simulink model "HybridControllerD3D3"  (Simulink 7.5)
settings: Solver=FixedStepDiscrete  StartTime=0.0  StopTime=inf  FixedStep=samplePeriod  RelTol=1e-3  AbsTol=1e-6
PreLoadFcn:
  | initializeSimulation;
InitFcn:
  | clear('all');
  | initializeSimulation;
undefined symbols (not defined in the file): damperA, damperB, damperC, damperCanon, DiscIntNeverNeededParam, flowCanon, forceCanon, frictionA, frictionB, frictionC, gasConstant, HybridCtrlParameters, lengthCanon, massA, massB, massC, massCanon, maxDisplA, maxDisplB, maxDisplC, maxOilVolume, maxVelocA, maxVelocB, maxVelocC, minDisplA, minDisplB, minDisplC, minVelocA, minVelocB, minVelocC, nAct, nAdcU, nDinp, nDout, nDucU, nEncU, precharge, pumpFlow, returnPress, staticForceA, staticForceB, staticForceC, supplyPress, velocCanon, volume, volumeCanon, yieldDisplA, yieldDisplB, yieldDisplC
libraries: simulink x2
(part 3 of 3)

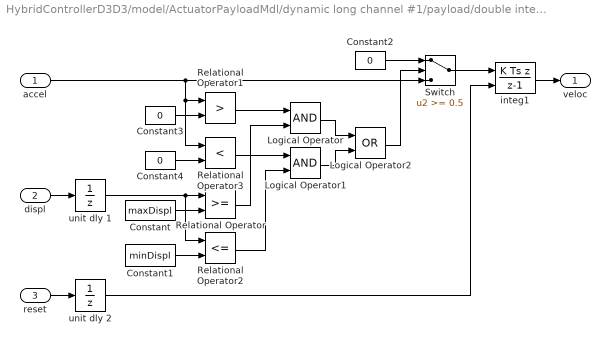
== system HybridControllerD3D3/model/ActuatorPayloadMdl/dynamic long channel #1/payload/double integrator/veloc gen ==
  accel : Inport  OutDataType=sfix(16)  OutScaling=2^0
  displ : Inport  Port=2  OutDataType=sfix(16)  OutScaling=2^0
  reset : Inport  Port=3  OutDataType=sfix(16)  OutScaling=2^0
  Constant : Constant  Value=maxDispl  OutDataType=sfix(16)  OutScaling=2^0
  Constant1 : Constant  Value=minDispl  OutDataType=sfix(16)  OutScaling=2^0
  Constant2 : Constant  Value=0  OutDataType=sfix(16)  OutScaling=2^0
  Constant3 : Constant  Value=0  OutDataType=sfix(16)  OutScaling=2^0
  Constant4 : Constant  Value=0  OutDataType=sfix(16)  OutScaling=2^0
  Logical Operator : Logic
  Logical Operator1 : Logic
  Logical Operator2 : Logic  Operator=OR
  Relational Operator : RelationalOperator  InputSameDT=on
  Relational Operator1 : RelationalOperator  Operator=>  InputSameDT=on
  Relational Operator2 : RelationalOperator  Operator=<=  InputSameDT=on
  Relational Operator3 : RelationalOperator  Operator=<  InputSameDT=on
  Switch : Switch  Threshold=0.5  SaturateOnIntegerOverflow=on  InputSameDT=on
  integ1 : DiscreteIntegrator  IntegratorMethod=Integration: Backward Euler  ExternalReset=either  SampleTime=-1  OutDataType=sfix(16)  OutScaling=2^0  LimitOutput=on  UpperSaturationLimit=maxVeloc  LowerSaturationLimit=minVeloc  ICPrevOutput=DiscIntNeverNeededParam  ICPrevScaledInput=DiscIntNeverNeededParam
  unit dly 1 : UnitDelay  SampleTime=-1
  unit dly 2 : UnitDelay  SampleTime=-1
  veloc : Outport  OutDataType=sfix(16)  OutScaling=2^0
  wires:
  unit dly 1/1 -> Relational Operator2/1, Relational Operator/1
  reset/1 -> unit dly 2/1
  displ/1 -> unit dly 1/1
  Logical Operator1/1 -> Logical Operator2/2
  unit dly 2/1 -> integ1/2
  Switch/1 -> integ1/1
  Logical Operator2/1 -> Switch/2
  Constant2/1 -> Switch/1
  Logical Operator/1 -> Logical Operator2/1
  Relational Operator3/1 -> Logical Operator1/1
  Constant4/1 -> Relational Operator3/2
  Relational Operator1/1 -> Logical Operator/1
  Constant3/1 -> Relational Operator1/2
  accel/1 -> Switch/3, Relational Operator1/1, Relational Operator3/1
  Constant1/1 -> Relational Operator2/2
  Relational Operator2/1 -> Logical Operator1/2
  Relational Operator/1 -> Logical Operator/2
  Constant/1 -> Relational Operator/2
  integ1/1 -> veloc/1

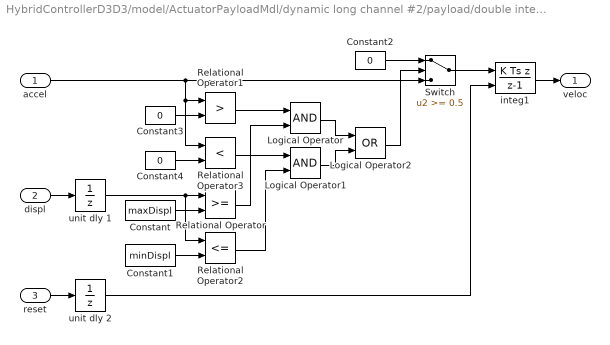
== system HybridControllerD3D3/model/ActuatorPayloadMdl/dynamic long channel #2/payload/double integrator/veloc gen ==
  accel : Inport  OutDataType=sfix(16)  OutScaling=2^0
  displ : Inport  Port=2  OutDataType=sfix(16)  OutScaling=2^0
  reset : Inport  Port=3  OutDataType=sfix(16)  OutScaling=2^0
  Constant : Constant  Value=maxDispl  OutDataType=sfix(16)  OutScaling=2^0
  Constant1 : Constant  Value=minDispl  OutDataType=sfix(16)  OutScaling=2^0
  Constant2 : Constant  Value=0  OutDataType=sfix(16)  OutScaling=2^0
  Constant3 : Constant  Value=0  OutDataType=sfix(16)  OutScaling=2^0
  Constant4 : Constant  Value=0  OutDataType=sfix(16)  OutScaling=2^0
  Logical Operator : Logic
  Logical Operator1 : Logic
  Logical Operator2 : Logic  Operator=OR
  Relational Operator : RelationalOperator  InputSameDT=on
  Relational Operator1 : RelationalOperator  Operator=>  InputSameDT=on
  Relational Operator2 : RelationalOperator  Operator=<=  InputSameDT=on
  Relational Operator3 : RelationalOperator  Operator=<  InputSameDT=on
  Switch : Switch  Threshold=0.5  SaturateOnIntegerOverflow=on  InputSameDT=on
  integ1 : DiscreteIntegrator  IntegratorMethod=Integration: Backward Euler  ExternalReset=either  SampleTime=-1  OutDataType=sfix(16)  OutScaling=2^0  LimitOutput=on  UpperSaturationLimit=maxVeloc  LowerSaturationLimit=minVeloc  ICPrevOutput=DiscIntNeverNeededParam  ICPrevScaledInput=DiscIntNeverNeededParam
  unit dly 1 : UnitDelay  SampleTime=-1
  unit dly 2 : UnitDelay  SampleTime=-1
  veloc : Outport  OutDataType=sfix(16)  OutScaling=2^0
  wires:
  unit dly 1/1 -> Relational Operator2/1, Relational Operator/1
  reset/1 -> unit dly 2/1
  displ/1 -> unit dly 1/1
  Logical Operator1/1 -> Logical Operator2/2
  unit dly 2/1 -> integ1/2
  Switch/1 -> integ1/1
  Logical Operator2/1 -> Switch/2
  Constant2/1 -> Switch/1
  Logical Operator/1 -> Logical Operator2/1
  Relational Operator3/1 -> Logical Operator1/1
  Constant4/1 -> Relational Operator3/2
  Relational Operator1/1 -> Logical Operator/1
  Constant3/1 -> Relational Operator1/2
  accel/1 -> Switch/3, Relational Operator1/1, Relational Operator3/1
  Constant1/1 -> Relational Operator2/2
  Relational Operator2/1 -> Logical Operator1/2
  Relational Operator/1 -> Logical Operator/2
  Constant/1 -> Relational Operator/2
  integ1/1 -> veloc/1

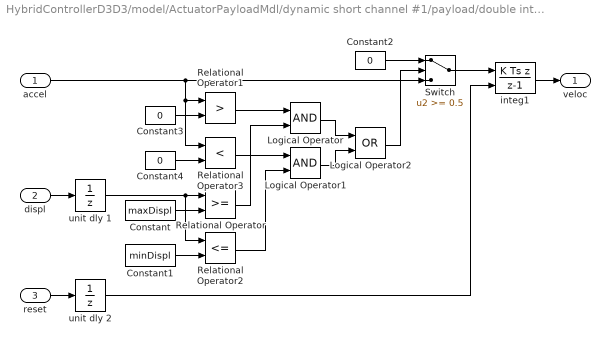
== system HybridControllerD3D3/model/ActuatorPayloadMdl/dynamic short channel #1/payload/double integrator/veloc gen ==
  accel : Inport  OutDataType=sfix(16)  OutScaling=2^0
  displ : Inport  Port=2  OutDataType=sfix(16)  OutScaling=2^0
  reset : Inport  Port=3  OutDataType=sfix(16)  OutScaling=2^0
  Constant : Constant  Value=maxDispl  OutDataType=sfix(16)  OutScaling=2^0
  Constant1 : Constant  Value=minDispl  OutDataType=sfix(16)  OutScaling=2^0
  Constant2 : Constant  Value=0  OutDataType=sfix(16)  OutScaling=2^0
  Constant3 : Constant  Value=0  OutDataType=sfix(16)  OutScaling=2^0
  Constant4 : Constant  Value=0  OutDataType=sfix(16)  OutScaling=2^0
  Logical Operator : Logic
  Logical Operator1 : Logic
  Logical Operator2 : Logic  Operator=OR
  Relational Operator : RelationalOperator  InputSameDT=on
  Relational Operator1 : RelationalOperator  Operator=>  InputSameDT=on
  Relational Operator2 : RelationalOperator  Operator=<=  InputSameDT=on
  Relational Operator3 : RelationalOperator  Operator=<  InputSameDT=on
  Switch : Switch  Threshold=0.5  SaturateOnIntegerOverflow=on  InputSameDT=on
  integ1 : DiscreteIntegrator  IntegratorMethod=Integration: Backward Euler  ExternalReset=either  SampleTime=-1  OutDataType=sfix(16)  OutScaling=2^0  LimitOutput=on  UpperSaturationLimit=maxVeloc  LowerSaturationLimit=minVeloc  ICPrevOutput=DiscIntNeverNeededParam  ICPrevScaledInput=DiscIntNeverNeededParam
  unit dly 1 : UnitDelay  SampleTime=-1
  unit dly 2 : UnitDelay  SampleTime=-1
  veloc : Outport  OutDataType=sfix(16)  OutScaling=2^0
  wires:
  unit dly 1/1 -> Relational Operator2/1, Relational Operator/1
  reset/1 -> unit dly 2/1
  displ/1 -> unit dly 1/1
  Logical Operator1/1 -> Logical Operator2/2
  unit dly 2/1 -> integ1/2
  Switch/1 -> integ1/1
  Logical Operator2/1 -> Switch/2
  Constant2/1 -> Switch/1
  Logical Operator/1 -> Logical Operator2/1
  Relational Operator3/1 -> Logical Operator1/1
  Constant4/1 -> Relational Operator3/2
  Relational Operator1/1 -> Logical Operator/1
  Constant3/1 -> Relational Operator1/2
  accel/1 -> Switch/3, Relational Operator1/1, Relational Operator3/1
  Constant1/1 -> Relational Operator2/2
  Relational Operator2/1 -> Logical Operator1/2
  Relational Operator/1 -> Logical Operator/2
  Constant/1 -> Relational Operator/2
  integ1/1 -> veloc/1

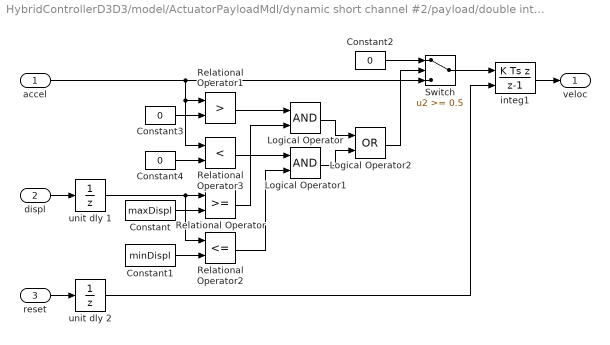
== system HybridControllerD3D3/model/ActuatorPayloadMdl/dynamic short channel #2/payload/double integrator/veloc gen ==
  accel : Inport  OutDataType=sfix(16)  OutScaling=2^0
  displ : Inport  Port=2  OutDataType=sfix(16)  OutScaling=2^0
  reset : Inport  Port=3  OutDataType=sfix(16)  OutScaling=2^0
  Constant : Constant  Value=maxDispl  OutDataType=sfix(16)  OutScaling=2^0
  Constant1 : Constant  Value=minDispl  OutDataType=sfix(16)  OutScaling=2^0
  Constant2 : Constant  Value=0  OutDataType=sfix(16)  OutScaling=2^0
  Constant3 : Constant  Value=0  OutDataType=sfix(16)  OutScaling=2^0
  Constant4 : Constant  Value=0  OutDataType=sfix(16)  OutScaling=2^0
  Logical Operator : Logic
  Logical Operator1 : Logic
  Logical Operator2 : Logic  Operator=OR
  Relational Operator : RelationalOperator  InputSameDT=on
  Relational Operator1 : RelationalOperator  Operator=>  InputSameDT=on
  Relational Operator2 : RelationalOperator  Operator=<=  InputSameDT=on
  Relational Operator3 : RelationalOperator  Operator=<  InputSameDT=on
  Switch : Switch  Threshold=0.5  SaturateOnIntegerOverflow=on  InputSameDT=on
  integ1 : DiscreteIntegrator  IntegratorMethod=Integration: Backward Euler  ExternalReset=either  SampleTime=-1  OutDataType=sfix(16)  OutScaling=2^0  LimitOutput=on  UpperSaturationLimit=maxVeloc  LowerSaturationLimit=minVeloc  ICPrevOutput=DiscIntNeverNeededParam  ICPrevScaledInput=DiscIntNeverNeededParam
  unit dly 1 : UnitDelay  SampleTime=-1
  unit dly 2 : UnitDelay  SampleTime=-1
  veloc : Outport  OutDataType=sfix(16)  OutScaling=2^0
  wires:
  unit dly 1/1 -> Relational Operator2/1, Relational Operator/1
  reset/1 -> unit dly 2/1
  displ/1 -> unit dly 1/1
  Logical Operator1/1 -> Logical Operator2/2
  unit dly 2/1 -> integ1/2
  Switch/1 -> integ1/1
  Logical Operator2/1 -> Switch/2
  Constant2/1 -> Switch/1
  Logical Operator/1 -> Logical Operator2/1
  Relational Operator3/1 -> Logical Operator1/1
  Constant4/1 -> Relational Operator3/2
  Relational Operator1/1 -> Logical Operator/1
  Constant3/1 -> Relational Operator1/2
  accel/1 -> Switch/3, Relational Operator1/1, Relational Operator3/1
  Constant1/1 -> Relational Operator2/2
  Relational Operator2/1 -> Logical Operator1/2
  Relational Operator/1 -> Logical Operator/2
  Constant/1 -> Relational Operator/2
  integ1/1 -> veloc/1

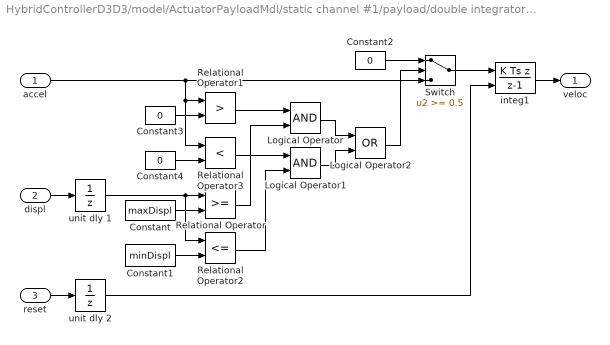
== system HybridControllerD3D3/model/ActuatorPayloadMdl/static channel #1/payload/double integrator/veloc gen ==
  accel : Inport  OutDataType=sfix(16)  OutScaling=2^0
  displ : Inport  Port=2  OutDataType=sfix(16)  OutScaling=2^0
  reset : Inport  Port=3  OutDataType=sfix(16)  OutScaling=2^0
  Constant : Constant  Value=maxDispl  OutDataType=sfix(16)  OutScaling=2^0
  Constant1 : Constant  Value=minDispl  OutDataType=sfix(16)  OutScaling=2^0
  Constant2 : Constant  Value=0  OutDataType=sfix(16)  OutScaling=2^0
  Constant3 : Constant  Value=0  OutDataType=sfix(16)  OutScaling=2^0
  Constant4 : Constant  Value=0  OutDataType=sfix(16)  OutScaling=2^0
  Logical Operator : Logic
  Logical Operator1 : Logic
  Logical Operator2 : Logic  Operator=OR
  Relational Operator : RelationalOperator  InputSameDT=on
  Relational Operator1 : RelationalOperator  Operator=>  InputSameDT=on
  Relational Operator2 : RelationalOperator  Operator=<=  InputSameDT=on
  Relational Operator3 : RelationalOperator  Operator=<  InputSameDT=on
  Switch : Switch  Threshold=0.5  SaturateOnIntegerOverflow=on  InputSameDT=on
  integ1 : DiscreteIntegrator  IntegratorMethod=Integration: Backward Euler  ExternalReset=either  SampleTime=-1  OutDataType=sfix(16)  OutScaling=2^0  LimitOutput=on  UpperSaturationLimit=maxVeloc  LowerSaturationLimit=minVeloc  ICPrevOutput=DiscIntNeverNeededParam  ICPrevScaledInput=DiscIntNeverNeededParam
  unit dly 1 : UnitDelay  SampleTime=-1
  unit dly 2 : UnitDelay  SampleTime=-1
  veloc : Outport  OutDataType=sfix(16)  OutScaling=2^0
  wires:
  unit dly 1/1 -> Relational Operator2/1, Relational Operator/1
  reset/1 -> unit dly 2/1
  displ/1 -> unit dly 1/1
  Logical Operator1/1 -> Logical Operator2/2
  unit dly 2/1 -> integ1/2
  Switch/1 -> integ1/1
  Logical Operator2/1 -> Switch/2
  Constant2/1 -> Switch/1
  Logical Operator/1 -> Logical Operator2/1
  Relational Operator3/1 -> Logical Operator1/1
  Constant4/1 -> Relational Operator3/2
  Relational Operator1/1 -> Logical Operator/1
  Constant3/1 -> Relational Operator1/2
  accel/1 -> Switch/3, Relational Operator1/1, Relational Operator3/1
  Constant1/1 -> Relational Operator2/2
  Relational Operator2/1 -> Logical Operator1/2
  Relational Operator/1 -> Logical Operator/2
  Constant/1 -> Relational Operator/2
  integ1/1 -> veloc/1

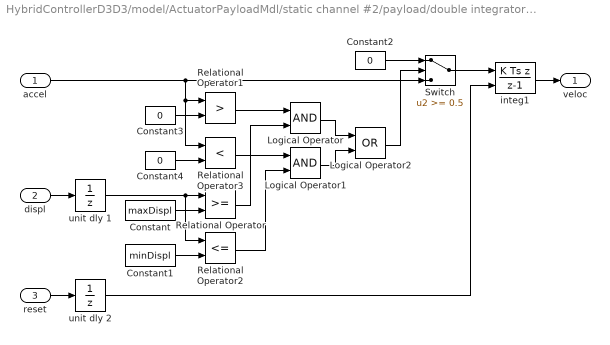
== system HybridControllerD3D3/model/ActuatorPayloadMdl/static channel #2/payload/double integrator/veloc gen ==
  accel : Inport  OutDataType=sfix(16)  OutScaling=2^0
  displ : Inport  Port=2  OutDataType=sfix(16)  OutScaling=2^0
  reset : Inport  Port=3  OutDataType=sfix(16)  OutScaling=2^0
  Constant : Constant  Value=maxDispl  OutDataType=sfix(16)  OutScaling=2^0
  Constant1 : Constant  Value=minDispl  OutDataType=sfix(16)  OutScaling=2^0
  Constant2 : Constant  Value=0  OutDataType=sfix(16)  OutScaling=2^0
  Constant3 : Constant  Value=0  OutDataType=sfix(16)  OutScaling=2^0
  Constant4 : Constant  Value=0  OutDataType=sfix(16)  OutScaling=2^0
  Logical Operator : Logic
  Logical Operator1 : Logic
  Logical Operator2 : Logic  Operator=OR
  Relational Operator : RelationalOperator  InputSameDT=on
  Relational Operator1 : RelationalOperator  Operator=>  InputSameDT=on
  Relational Operator2 : RelationalOperator  Operator=<=  InputSameDT=on
  Relational Operator3 : RelationalOperator  Operator=<  InputSameDT=on
  Switch : Switch  Threshold=0.5  SaturateOnIntegerOverflow=on  InputSameDT=on
  integ1 : DiscreteIntegrator  IntegratorMethod=Integration: Backward Euler  ExternalReset=either  SampleTime=-1  OutDataType=sfix(16)  OutScaling=2^0  LimitOutput=on  UpperSaturationLimit=maxVeloc  LowerSaturationLimit=minVeloc  ICPrevOutput=DiscIntNeverNeededParam  ICPrevScaledInput=DiscIntNeverNeededParam
  unit dly 1 : UnitDelay  SampleTime=-1
  unit dly 2 : UnitDelay  SampleTime=-1
  veloc : Outport  OutDataType=sfix(16)  OutScaling=2^0
  wires:
  unit dly 1/1 -> Relational Operator2/1, Relational Operator/1
  reset/1 -> unit dly 2/1
  displ/1 -> unit dly 1/1
  Logical Operator1/1 -> Logical Operator2/2
  unit dly 2/1 -> integ1/2
  Switch/1 -> integ1/1
  Logical Operator2/1 -> Switch/2
  Constant2/1 -> Switch/1
  Logical Operator/1 -> Logical Operator2/1
  Relational Operator3/1 -> Logical Operator1/1
  Constant4/1 -> Relational Operator3/2
  Relational Operator1/1 -> Logical Operator/1
  Constant3/1 -> Relational Operator1/2
  accel/1 -> Switch/3, Relational Operator1/1, Relational Operator3/1
  Constant1/1 -> Relational Operator2/2
  Relational Operator2/1 -> Logical Operator1/2
  Relational Operator/1 -> Logical Operator/2
  Constant/1 -> Relational Operator/2
  integ1/1 -> veloc/1

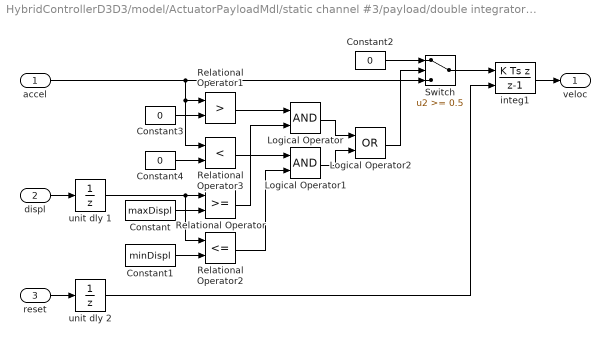
== system HybridControllerD3D3/model/ActuatorPayloadMdl/static channel #3/payload/double integrator/veloc gen ==
  accel : Inport  OutDataType=sfix(16)  OutScaling=2^0
  displ : Inport  Port=2  OutDataType=sfix(16)  OutScaling=2^0
  reset : Inport  Port=3  OutDataType=sfix(16)  OutScaling=2^0
  Constant : Constant  Value=maxDispl  OutDataType=sfix(16)  OutScaling=2^0
  Constant1 : Constant  Value=minDispl  OutDataType=sfix(16)  OutScaling=2^0
  Constant2 : Constant  Value=0  OutDataType=sfix(16)  OutScaling=2^0
  Constant3 : Constant  Value=0  OutDataType=sfix(16)  OutScaling=2^0
  Constant4 : Constant  Value=0  OutDataType=sfix(16)  OutScaling=2^0
  Logical Operator : Logic
  Logical Operator1 : Logic
  Logical Operator2 : Logic  Operator=OR
  Relational Operator : RelationalOperator  InputSameDT=on
  Relational Operator1 : RelationalOperator  Operator=>  InputSameDT=on
  Relational Operator2 : RelationalOperator  Operator=<=  InputSameDT=on
  Relational Operator3 : RelationalOperator  Operator=<  InputSameDT=on
  Switch : Switch  Threshold=0.5  SaturateOnIntegerOverflow=on  InputSameDT=on
  integ1 : DiscreteIntegrator  IntegratorMethod=Integration: Backward Euler  ExternalReset=either  SampleTime=-1  OutDataType=sfix(16)  OutScaling=2^0  LimitOutput=on  UpperSaturationLimit=maxVeloc  LowerSaturationLimit=minVeloc  ICPrevOutput=DiscIntNeverNeededParam  ICPrevScaledInput=DiscIntNeverNeededParam
  unit dly 1 : UnitDelay  SampleTime=-1
  unit dly 2 : UnitDelay  SampleTime=-1
  veloc : Outport  OutDataType=sfix(16)  OutScaling=2^0
  wires:
  unit dly 1/1 -> Relational Operator2/1, Relational Operator/1
  reset/1 -> unit dly 2/1
  displ/1 -> unit dly 1/1
  Logical Operator1/1 -> Logical Operator2/2
  unit dly 2/1 -> integ1/2
  Switch/1 -> integ1/1
  Logical Operator2/1 -> Switch/2
  Constant2/1 -> Switch/1
  Logical Operator/1 -> Logical Operator2/1
  Relational Operator3/1 -> Logical Operator1/1
  Constant4/1 -> Relational Operator3/2
  Relational Operator1/1 -> Logical Operator/1
  Constant3/1 -> Relational Operator1/2
  accel/1 -> Switch/3, Relational Operator1/1, Relational Operator3/1
  Constant1/1 -> Relational Operator2/2
  Relational Operator2/1 -> Logical Operator1/2
  Relational Operator/1 -> Logical Operator/2
  Constant/1 -> Relational Operator/2
  integ1/1 -> veloc/1

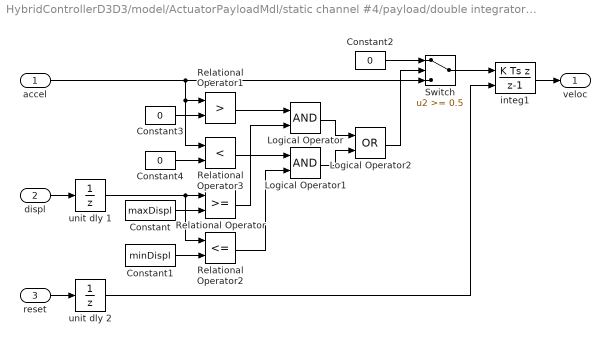
== system HybridControllerD3D3/model/ActuatorPayloadMdl/static channel #4/payload/double integrator/veloc gen ==
  accel : Inport  OutDataType=sfix(16)  OutScaling=2^0
  displ : Inport  Port=2  OutDataType=sfix(16)  OutScaling=2^0
  reset : Inport  Port=3  OutDataType=sfix(16)  OutScaling=2^0
  Constant : Constant  Value=maxDispl  OutDataType=sfix(16)  OutScaling=2^0
  Constant1 : Constant  Value=minDispl  OutDataType=sfix(16)  OutScaling=2^0
  Constant2 : Constant  Value=0  OutDataType=sfix(16)  OutScaling=2^0
  Constant3 : Constant  Value=0  OutDataType=sfix(16)  OutScaling=2^0
  Constant4 : Constant  Value=0  OutDataType=sfix(16)  OutScaling=2^0
  Logical Operator : Logic
  Logical Operator1 : Logic
  Logical Operator2 : Logic  Operator=OR
  Relational Operator : RelationalOperator  InputSameDT=on
  Relational Operator1 : RelationalOperator  Operator=>  InputSameDT=on
  Relational Operator2 : RelationalOperator  Operator=<=  InputSameDT=on
  Relational Operator3 : RelationalOperator  Operator=<  InputSameDT=on
  Switch : Switch  Threshold=0.5  SaturateOnIntegerOverflow=on  InputSameDT=on
  integ1 : DiscreteIntegrator  IntegratorMethod=Integration: Backward Euler  ExternalReset=either  SampleTime=-1  OutDataType=sfix(16)  OutScaling=2^0  LimitOutput=on  UpperSaturationLimit=maxVeloc  LowerSaturationLimit=minVeloc  ICPrevOutput=DiscIntNeverNeededParam  ICPrevScaledInput=DiscIntNeverNeededParam
  unit dly 1 : UnitDelay  SampleTime=-1
  unit dly 2 : UnitDelay  SampleTime=-1
  veloc : Outport  OutDataType=sfix(16)  OutScaling=2^0
  wires:
  unit dly 1/1 -> Relational Operator2/1, Relational Operator/1
  reset/1 -> unit dly 2/1
  displ/1 -> unit dly 1/1
  Logical Operator1/1 -> Logical Operator2/2
  unit dly 2/1 -> integ1/2
  Switch/1 -> integ1/1
  Logical Operator2/1 -> Switch/2
  Constant2/1 -> Switch/1
  Logical Operator/1 -> Logical Operator2/1
  Relational Operator3/1 -> Logical Operator1/1
  Constant4/1 -> Relational Operator3/2
  Relational Operator1/1 -> Logical Operator/1
  Constant3/1 -> Relational Operator1/2
  accel/1 -> Switch/3, Relational Operator1/1, Relational Operator3/1
  Constant1/1 -> Relational Operator2/2
  Relational Operator2/1 -> Logical Operator1/2
  Relational Operator/1 -> Logical Operator/2
  Constant/1 -> Relational Operator/2
  integ1/1 -> veloc/1

== stateflow chart model/simPC HC/Predictor-Corrector ==
  state HybridController [parallel]
    settings: executionOrder=1
    state Predict
      en: state = 1;
      en: setCurDsp(com,i/N);
      en: diSD = 1;
      en: i = 1; iSD = 0;
      en: predictD3(com,i/N);
      du: i++;
      du: predictD3(com,i/N);
    state Initialize
      en: i = 1; iSD = 0;
      en: diSD = 1;
      en: initData(nAct,dtCon);
      en: zeroDsp(com);
    state AutoSlowDown
      en: state = 2;
      en: diSD = 4-i/(0.2*N);
      en: i += diSD; iSD = i;
      en: predictD3(com,i/N);
      du: diSD = 4-i/(0.2*N);
      du: i += diSD; iSD = i;
      du: predictD3(com,i/N);
    state Correct
      en: state = 0;
      en: setCurDsp(com,i/N);
      en: dspLocal = dsp; setNewDsp(dspLocal);
      en: di = min(max(diSD+1/(0.2*N)*(i-iSD),0.001),1.0);
      en: i = min(i+di,N);
      en: correctD3(com,i/N);
      du: di = min(max(diSD+1/(0.2*N)*(i-iSD),0.001),1.0);
      du: i = min(i+di,N);
      du: correctD3(com,i/N);
    Correct -> Predict : [i>=N]
    (default) -> Initialize
    Predict -> Correct [order 2] : [flag==1]
    Initialize -> Correct : [flag==1]
    AutoSlowDown -> Correct : [flag==1]
    Predict -> AutoSlowDown [order 1] : [i>=0.6*N && flag~=1]
  data: dsp input double size=nAct+1; flag input double size=1; com output double size=nAct+1; state output double size=1; i output double size=1; N local double size=1; nAct parameter double size=1 =1; di local double size=1; diSD local double size=1; iSD local double size=1; dspLocal local double size=nAct+1
